simulink model "LQG"  (R2020a)
settings: Solver=VariableStepAuto  StartTime=0.0  StopTime=10.0  RelTol=1e-3
PreLoadFcn:
  | kalman_params
values from neighbouring files (symbols this model uses):
  A = [0, 1; 4.1*10^4, 0]    [kalman_params.m]
  B = [0; -9.12]    [kalman_params.m]
  C = [1 0;0 1]    [kalman_params.m]
  D = [0; 0]    [kalman_params.m]
  sysKF = ss(A-Kf*C, [B Kf], eye(2), 0*[B Kf])    [kalman_params.m]
undefined symbols (not defined in the file or in its folder): Kc
settings Model: Creator=prans  LastModifiedBy=prans

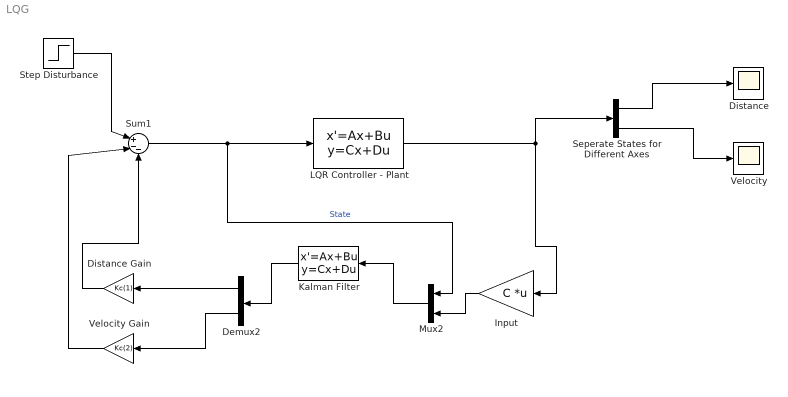
== system LQG ==
  Demux2 : Demux  Outputs=2
  Distance : Scope
  Distance Gain : Gain  Gain=Kc(1)
  Input : Gain  Gain=C  Multiplication=Matrix(K*u) (u vector)
  Kalman Filter : StateSpace  A=sysKF.a  B=sysKF.b  C=sysKF.c  D=sysKF.d  InitialCondition=[1 0]
  LQR Controller - Plant : StateSpace  A=A  B=B  C=C  D=D  InitialCondition=[1 0]
  Mux2 : Mux  Inputs=2
  Seperate States for Different Axes : Demux  Outputs=2
  Step Disturbance : Step  Time=0  After=0  SampleTime=0
  Sum1 : Sum  Inputs=|+--
  Velocity : Scope
  Velocity Gain : Gain  Gain=Kc(2)
  wires:
  Demux2/1 -> Distance Gain/1
  Mux2/1 -> Kalman Filter/1
  Input/1 -> Mux2/2
  Kalman Filter/1 -> Demux2/1
  LQR Controller - Plant/1 -> Input/1, Seperate States for Different Axes/1
  Seperate States for Different Axes/2 -> Velocity/1
  Sum1/1 -> Mux2/1, LQR Controller - Plant/1  "State"
  Distance Gain/1 -> Sum1/3
  Seperate States for Different Axes/1 -> Distance/1
  Demux2/2 -> Velocity Gain/1
  Velocity Gain/1 -> Sum1/2
  Step Disturbance/1 -> Sum1/1
